simulink model "Merger"  (R2021a)
settings: Solver=FixedStepAuto  StartTime=0.0  StopTime=Inf  RelTol=1e-5
model workspace (MAT data in the model file):
  RefVel = 0.1
values from neighbouring files (symbols this model uses):
  waypoints = waypoints(:,1:2)    [setup.m]    (also in waypoint_genearator.m)
libraries: visionsinks x4, drivingvehiclecontroller x1, robotalgslib x1
settings Model: PauseTimes=0  Creator=darks  LastModifiedBy=Avvienash
settings DebuggingCC: SFMachineParentedDataDiag=warning
settings SFSimCC: CustomCodeUndefinedFunction=UseInterfaceOnly

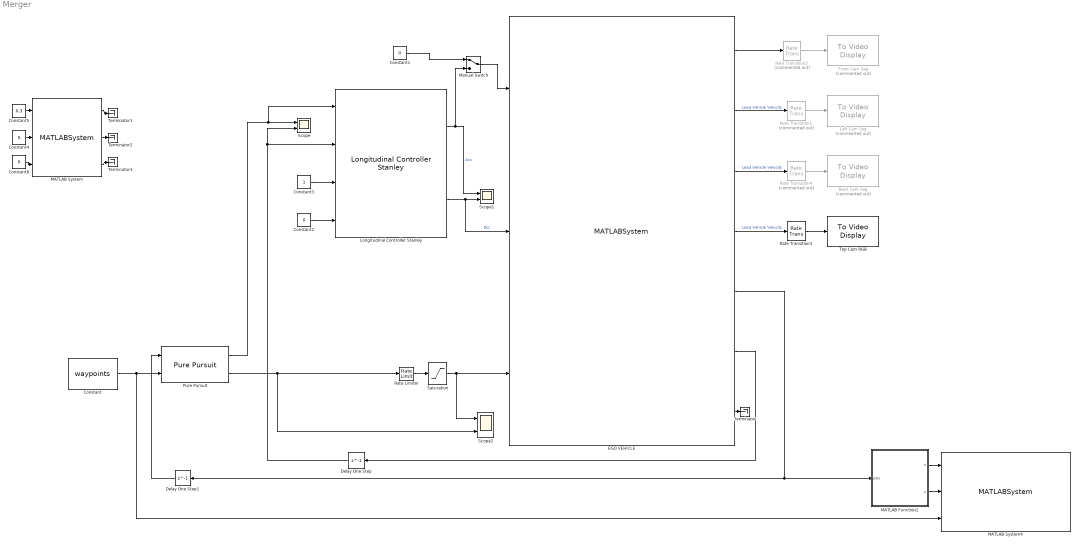
== system Merger ==
  Back Cam Seg : visionsinks/To Video Display  Commented=on  windowSizeMode=Normal  openAtMdlStart=on  fullScreen=off  videoWindowX=59  videoWindowY=827  saveWindowSize=off  videoWindowWidth=1167  videoWindowHeight=655  inputColorFormat=RGB  inputType=Obsolete  imagePorts=One multidimensional signal  OutputDevice=On-screen video monitor  dataOrg=Column-major  isWindowOpen=off
  Constant : Constant  Value=waypoints
  Constant{1..2,4,6} (4 alike) : Constant  Value=0
  Constant3 : Constant
  Constant5 : Constant  Value=0.3
  Delay One Step : Delay  DelayLength=1
  Delay One Step1 : Delay  DelayLength=1  InitialCondition=[150 -1.5 2.61799]
  EGO VEHICLE : MATLABSystem  System=merger  SimulateUsing=Interpreted execution
      mask Type: merger
      mask Display:
      | disp('merger');
      | port_label('input',1,'throttle');
      | port_label('input',2,'brake');
      | port_label('input',3,'steer');
      | port_label('output',1,'FRONT_CAM_SEG');
      | port_label('output',2,'LEFT_CAM_SEG');
      | port_label('output',3,'BACK_CAM_SEG');
      | port_label('output',4,'TOP_CAM_RGB');
      | port_label('output',5,'pos');
      | port_label('output',6,'long_velocity');
      | port_label('output',7,'ang_velocity');
  Front Cam Seg : visionsinks/To Video Display  Commented=on  windowSizeMode=Normal  openAtMdlStart=on  fullScreen=off  videoWindowX=0  videoWindowY=34  saveWindowSize=off  videoWindowWidth=2560  videoWindowHeight=1494  inputColorFormat=RGB  inputType=Obsolete  imagePorts=One multidimensional signal  OutputDevice=On-screen video monitor  dataOrg=Column-major  isWindowOpen=off
  Left Cam Seg : visionsinks/To Video Display  Commented=on  windowSizeMode=Normal  openAtMdlStart=on  fullScreen=off  videoWindowX=0  videoWindowY=34  saveWindowSize=off  videoWindowWidth=2560  videoWindowHeight=1494  inputColorFormat=RGB  inputType=Obsolete  imagePorts=One multidimensional signal  OutputDevice=On-screen video monitor  dataOrg=Column-major  isWindowOpen=off
  Longitudinal Controller Stanley : drivingvehiclecontroller/Longitudinal Controller Stanley  Kp=0.2  Ki=0.9  SampleTime=0.05  MaxAcceleration=1  MaxDeceleration=1
      settings: SourceProductBaseCode=DR
  MATLAB Function2 : MATLAB Function  TreatAsAtomicUnit=on
  MATLAB System : MATLABSystem  System=NPC2  SimulateUsing=Interpreted execution
      mask Type: NPC2
      mask Display:
      | disp('NPC2');
      | port_label('input',1,'throttle');
      | port_label('input',2,'brake');
      | port_label('input',3,'steer');
      | port_label('output',1,'pos');
      | port_label('output',2,'long_velocity');
      | port_label('output',3,'ang_velocity');
  MATLAB System4 : MATLABSystem  System=traffic_view  SimulateUsing=Interpreted execution
      mask Type: traffic_view
      mask Display:
      | disp('traffic_view');
      | port_label('input',1,'x');
      | port_label('input',2,'y');
      | port_label('input',3,'waypoints');
  Manual Switch : ManualSwitch
  Pure Pursuit : robotalgslib/Pure Pursuit  DesiredLinearVelocity=5  MaxAngularVelocity=1  LookaheadDistance=5  TargetDirPort=off  SimulateUsing=Code generation
  Rate Limiter : RateLimiter  SampleTimeMode=inherited
  Rate Transition1 : RateTransition  Commented=on  OutPortSampleTime=.1
  Rate Transition2 : RateTransition  Commented=on  OutPortSampleTime=.1
  Rate Transition3 : RateTransition  OutPortSampleTime=.1
  Rate Transition4 : RateTransition  Commented=on  OutPortSampleTime=.1
  Saturation : Saturate  UpperLimit=1  LowerLimit=-1
  Scope : Scope  NumInputPorts=2
  Scope1 : Scope  NumInputPorts=2
  Scope2 : Scope  NumInputPorts=2
  Terminator{,1..3} (4 alike) : Terminator
  Top Cam RGB : visionsinks/To Video Display  windowSizeMode=True size (1:1)  openAtMdlStart=on  fullScreen=off  videoWindowX=293  videoWindowY=157  saveWindowSize=off  videoWindowWidth=1920  videoWindowHeight=540  inputColorFormat=RGB  inputType=Obsolete  imagePorts=One multidimensional signal  OutputDevice=On-screen video monitor  dataOrg=Column-major  isWindowOpen=off
  wires:
  Rate Transition2/1 -> Front Cam Seg/1
  Rate Transition1/1 -> Left Cam Seg/1
  EGO VEHICLE/1 -> Rate Transition2/1
  EGO VEHICLE/2 -> Rate Transition1/1  "Lead Vehicle Velocity"
  Constant2/1 -> Longitudinal Controller Stanley/4
  Constant3/1 -> Longitudinal Controller Stanley/3
  Longitudinal Controller Stanley/1 -> Manual Switch/2, Scope1/1  "Acc"
  Longitudinal Controller Stanley/2 -> Scope1/2, EGO VEHICLE/2  "Dcc"
  Delay One Step/1 -> Longitudinal Controller Stanley/2, Scope/2
  Constant/1 -> MATLAB System4/3, Pure Pursuit/2
  EGO VEHICLE/5 -> MATLAB Function2/1(pos), Delay One Step1/1
  Delay One Step1/1 -> Pure Pursuit/1
  EGO VEHICLE/6 -> Delay One Step/1
  Pure Pursuit/1 -> Scope/1, Longitudinal Controller Stanley/1
  MATLAB Function2/2(y) -> MATLAB System4/2
  MATLAB Function2/1(x) -> MATLAB System4/1
  Saturation/1 -> Scope2/1, EGO VEHICLE/3
  Pure Pursuit/2 -> Scope2/2, Rate Limiter/1
  Rate Limiter/1 -> Saturation/1
  EGO VEHICLE/7 -> Terminator/1
  EGO VEHICLE/4 -> Rate Transition3/1  "Lead Vehicle Velocity"
  Rate Transition3/1 -> Top Cam RGB/1
  EGO VEHICLE/3 -> Rate Transition4/1  "Lead Vehicle Velocity"
  Rate Transition4/1 -> Back Cam Seg/1
  Constant1/1 -> Manual Switch/1
  Manual Switch/1 -> EGO VEHICLE/1
  Constant4/1 -> MATLAB System/2
  Constant5/1 -> MATLAB System/1
  Constant6/1 -> MATLAB System/3
  MATLAB System/1 -> Terminator1/1
  MATLAB System/2 -> Terminator2/1
  MATLAB System/3 -> Terminator3/1

== matlab function Merger/MATLAB Function2 ==
  data: x output; pos input; y output
function [x,y] = xy(pos)

	x = pos(1);
    y = pos(2);
end
